simulink model "SIMULINK_01_PARAMETRIC_IDENTIFICATION"  (R2020a)
settings: Solver=FixedStepAuto  StartTime=0.0  StopTime=10  FixedStep=0.001  RelTol=1e-3
settings Model: Creator=alejandropuerta  LastModifiedBy=USUARIO

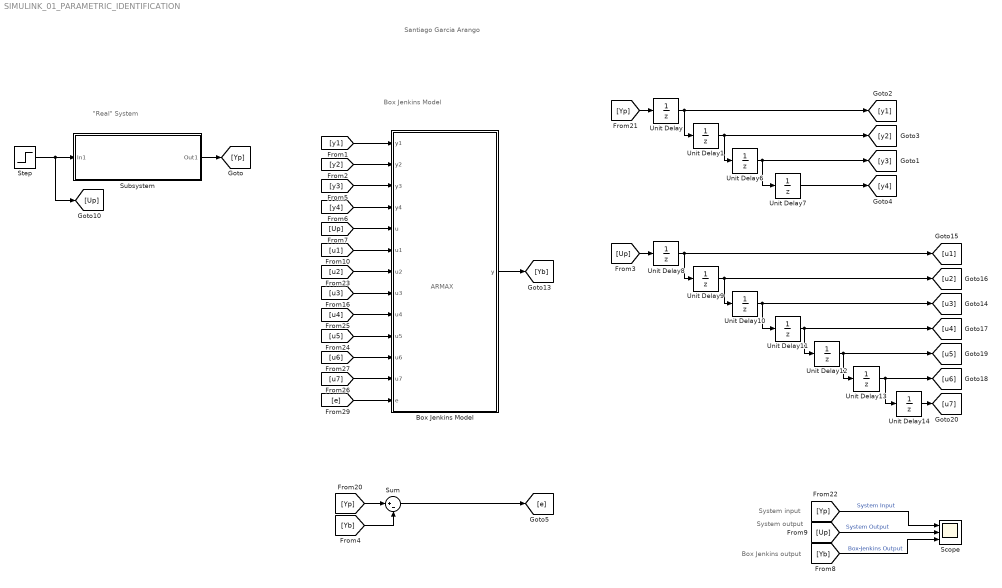
== system SIMULINK_01_PARAMETRIC_IDENTIFICATION ==
  note: Santiago Garcia Arango
  note: Box Jenkins Model
  note: ARMAX
  note: "Real" System
  note: Box Jenkins output
  note: System input
  note: System output
  Box Jenkins Model : MATLAB Function  TreatAsAtomicUnit=on
  Scope : Scope  NumInputPorts=3
  Step : Step  Before=1  After=0  SampleTime=0.001
  Subsystem : Subsystem
  Sum : Sum  Inputs=|+-
  Unit Delay{,1,6..14} (11 alike) : UnitDelay  SampleTime=-1  HasFrameUpgradeWarning=on
  wires:
  Subsystem/1(Out1) -> [Yp]
  Step/1 -> [Up], Subsystem/1(In1)
  Box Jenkins Model/1(y) -> [Yb]
  Unit Delay/1 -> [y1], Unit Delay1/1
  Unit Delay1/1 -> [y2], Unit Delay6/1
  [y1] -> Box Jenkins Model/1(y1)
  [y2] -> Box Jenkins Model/2(y2)
  [Yb] -> Sum/2
  Sum/1 -> [e]
  [Yp] -> Sum/1
  [Yp] -> Unit Delay/1
  [Up] -> Scope/2  "System Output"
  [Yp] -> Scope/1  "System Input"
  [Yb] -> Scope/3  "Box-Jenkins Output"
  Unit Delay6/1 -> [y3], Unit Delay7/1
  Unit Delay7/1 -> [y4]
  Unit Delay8/1 -> [u1], Unit Delay9/1
  Unit Delay10/1 -> [u3], Unit Delay11/1
  Unit Delay9/1 -> [u2], Unit Delay10/1
  [Up] -> Unit Delay8/1
  Unit Delay11/1 -> Unit Delay12/1, [u4]
  Unit Delay12/1 -> [u5], Unit Delay13/1
  Unit Delay13/1 -> Unit Delay14/1, [u6]
  Unit Delay14/1 -> [u7]
  [y3] -> Box Jenkins Model/3(y3)
  [y4] -> Box Jenkins Model/4(y4)
  [Up] -> Box Jenkins Model/5(u)
  [u1] -> Box Jenkins Model/6(u1)
  [u2] -> Box Jenkins Model/7(u2)
  [u3] -> Box Jenkins Model/8(u3)
  [u4] -> Box Jenkins Model/9(u4)
  [u5] -> Box Jenkins Model/10(u5)
  [u6] -> Box Jenkins Model/11(u6)
  [u7] -> Box Jenkins Model/12(u7)
  [e] -> Box Jenkins Model/13(e)

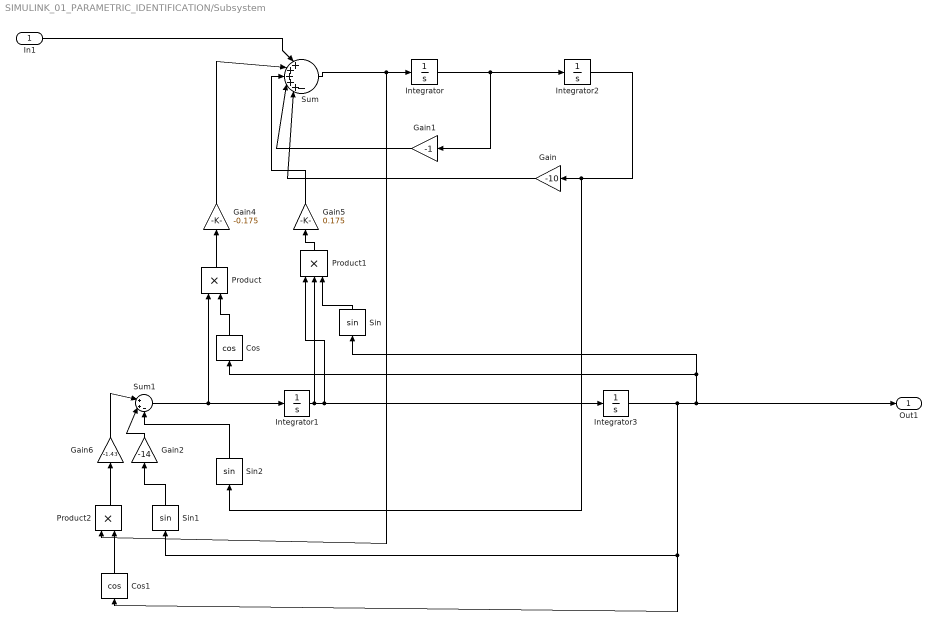
== system SIMULINK_01_PARAMETRIC_IDENTIFICATION/Subsystem ==
  In1 : Inport
  Cos : Trigonometry  Operator=cos
  Cos1 : Trigonometry  Operator=cos
  Gain : Gain  Gain=-10
  Gain1 : Gain  Gain=-1
  Gain2 : Gain  Gain=-14
  Gain4 : Gain  Gain=-0.175
  Gain5 : Gain  Gain=0.175
  Gain6 : Gain  Gain=-1.43
  Integrator{,1..3} (4 alike) : Integrator
  Product : Product
  Product1 : Product  Inputs=3
  Product2 : Product
  Sin : Trigonometry
  Sin1 : Trigonometry
  Sin2 : Trigonometry
  Sum : Sum  Inputs=|+++++-
  Sum1 : Sum  Inputs=|++-
  Out1 : Outport  VectorParamsAs1DForOutWhenUnconnected=off
  wires:
  Gain2/1 -> Sum1/2
  Gain6/1 -> Sum1/1
  Sin2/1 -> Sum1/3
  Integrator1/1 -> Integrator3/1, Product1/1, Product1/2
  Cos1/1 -> Product2/2
  Gain/1 -> Sum/5
  Integrator2/1 -> Sin2/1, Gain/1
  Gain5/1 -> Sum/3
  Product1/1 -> Gain5/1
  Gain1/1 -> Sum/4
  In1/1 -> Sum/1
  Sum1/1 -> Product/1, Integrator1/1
  Integrator3/1 -> Sin1/1, Cos1/1, Out1/1, Cos/1, Sin/1
  Product2/1 -> Gain6/1
  Gain4/1 -> Sum/2
  Product/1 -> Gain4/1
  Sin1/1 -> Gain2/1
  Sin/1 -> Product1/3
  Integrator/1 -> Gain1/1, Integrator2/1
  Cos/1 -> Product/2
  Sum/1 -> Product2/1, Integrator/1

== matlab function SIMULINK_01_PARAMETRIC_IDENTIFICATION/Box Jenkins Model ==
  data: y1 input; y2 input; y3 input; y4 input; u input; u1 input; u2 input; u3 input; u4 input; u5 input; u6 input; u7 input; y output; e input
function y = fcn(y1,y2,y3,y4,u,u1,u2,u3,u4,u5,u6,u7,e)

a1 = 3.999;
a2 = -5.996;
a3 = 3.996;
a4 = -0.9987;
b0 = -1.14e-12;
b1 = 1.754e-15;
b2 = 1.851e-15;
b3 = -9.474e-07;
b4 = 9.479e-07;
b5 = 9.465e-07;
b6 = -9.47e-07;
b7 = 1.623e-14;

y = a1*y1+a2*y2+a3*y3+a4*y4+b0*u+b1*u1+b2*u2+b3*u3+b4*u4+b5*u5+b6*u6+b7*u7+e;
